simulink model "flight_sim"  (R2021b)
settings: Solver=ode45  StartTime=0.0  StopTime=300  RelTol=1e-3
values from neighbouring files (symbols this model uses):
  fpa_0 = pi/2    (= 1.57079632679)    [Falcon_1_para.m]
  fpa_in = 0.10    (= 0.1)    [Falcon_1_para.m]
  g = 9.81    [Falcon_1_para.m]
  h_0 = 0    [Falcon_1_para.m]
  m_dot = 132.46    [Falcon_1_para.m]
  m_zfw = m_pay + m_dry    (= 6360.7)    [Falcon_1_para.m]
  R_E = 6731e03    (= 6731000)    [Falcon_1_para.m]
  t_turn = 30.0    (= 30)    [Falcon_1_para.m]
  v_0 = 0.01    [Falcon_1_para.m]
  x_0 = 0    [Falcon_1_para.m]
undefined symbols (not defined in the file or in its folder): Earth, WGS84
libraries: aerolibfltsims x2, slpidlib x1, aerolibtransform2 x1, simulink x1
settings Model: Creator=hashi  LastModifiedBy=hashi

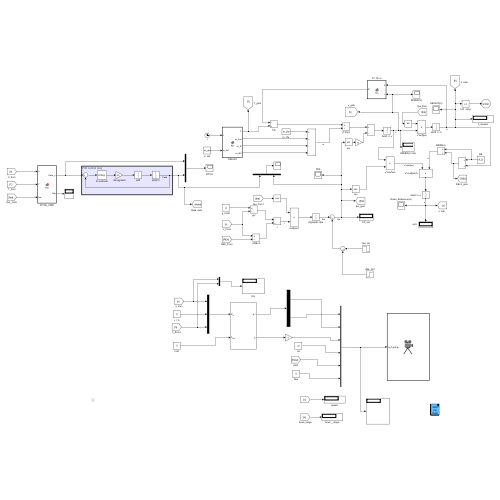
[thumbnail: Simulink's stored preview of the top-level diagram]
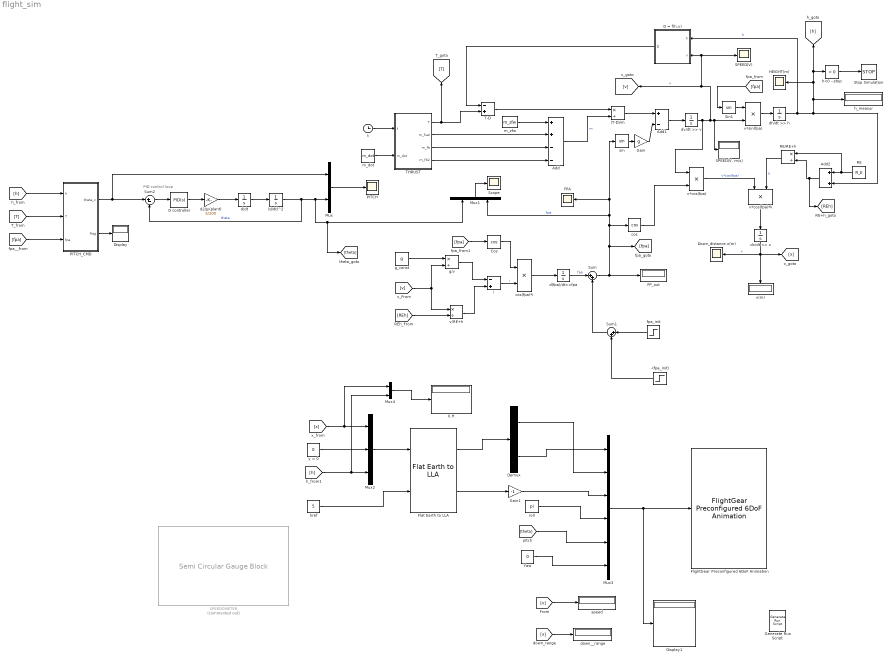
== system flight_sim ==
  note: PID control loop
  (T-D)/m : Product  Inputs=*/
  (d/dt)^2 : Integrator  InitialCondition=pi/2
  -(fpa_init) : Step  Time=t_turn+1  Before=-fpa_in  After=-fpa_in  SampleTime=0
  Add : Sum  Inputs=++--
  Add1 : Sum  Inputs=+-
  Add2 : Sum
  Cos : Trigonometry  Operator=cos
  D = f(h,v) : MATLAB Function  TreatAsAtomicUnit=on
  D controller : slpidlib/PID Controller  Controller=PID  Form=Parallel  TimeDomain=Continuous-time  UseExternalTs=off  SampleTime=-1  IntegratorMethod=Forward Euler  FilterMethod=Forward Euler  ControllerParametersSource=internal  P=0  I=0  D=200/5  UseFilter=on  N=100  TunerSelectOption=Transfer Function Based (PID Tuner App)  InitialConditionSource=internal  InitialConditionForIntegrator=0  InitialConditionForFilter=0  DifferentiatorICPrevScaledInput=0  ExternalReset=none  TrackingMode=off  Kt=1  LimitOutput=off  SatLimitsSource=internal  UpperSaturationLimit=inf  LowerSaturationLimit=-inf  LinearizeAsGain=on  AntiWindupMode=none  Kb=1  POutMin=[]  POutMax=[]  IOutMin=[]  IOutMax=[]  DOutMin=[]  DOutMax=[]  NOutMin=[]  NOutMax=[]  SumOutMin=[]  SumOutMax=[]  SaturationOutMin=[]  SaturationOutMax=[]  PParamMin=[]  PParamMax=[]  IParamMin=[]  IParamMax=[]  DParamMin=[]  DParamMax=[]  NParamMin=[]  NParamMax=[]  KbParamMin=[]  KbParamMax=[]  KtParamMin=[]  KtParamMax=[]  KbOutMin=[]  KbOutMax=[]  KtOutMin=[]  KtOutMax=[]  IntegratorOutMin=[]  IntegratorOutMax=[]  FilterOutMin=[]  FilterOutMax=[]  SumI1OutMin=[]  SumI1OutMax=[]  SumI2OutMin=[]  SumI2OutMax=[]  SumI3OutMin=[]  SumI3OutMax=[]  SumI4OutMin=[]  SumI4OutMax=[]  SumDOutMin=[]  SumDOutMax=[]  DifferentiatorOutMin=[]  DifferentiatorOutMax=[]  FilterDiffOutCoefMin=[]  FilterDiffOutCoefMax=[]  ReciprocalOutMin=[]  ReciprocalOutMax=[]  SumDenOutMin=[]  SumDenOutMax=[]  SumNumOutMin=[]  SumNumOutMax=[]  DivideOutMin=[]  DivideOutMax=[]  UdiffTsProdOutMin=[]  UdiffTsProdOutMax=[]  NTsProdOutMin=[]  NTsProdOutMax=[]  UintegralTsProdOutMin=[]  UintegralTsProdOutMax=[]  UngainTsProdOutMin=[]  UngainTsProdOutMax=[]  IntegratorContinuousStateAttributes=''  IntegratorStateMustResolveToSignalObject=off  IntegratorRTWStateStorageClass=Auto  FilterContinuousStateAttributes=''  FilterStateMustResolveToSignalObject=off  FilterRTWStateStorageClass=Auto  ParallelPVariant=InternalParameters  IdealPVariant=Disabled  IVariant=InternalParameters  DVariant=InternalParameters  IntegratorVariant=Continuous  SatVariant=Disabled  AWVariant=Passthrough  PCopyVariant=Disabled  TRVariant=Disabled  FdbkBlocksVariant=Forward  IdealPFdbkVariant=Disabled  SatFdbkVariant=Disabled  DerivativeFilterVariant=ContFilter  NVariant=InternalParameters  NCopyVariant=Disabled  FilterICVariant=InternalICsFilter  IntegratorICVariant=InternalICs  ExternalResetVariant=Disabled  TRSumVariant=Passthrough  SumFdbkVariant=Disabled  SumVariant=Sum_PID  TsampFilterVariant=InternalTs  TsampNgainVariant=Passthrough  TsampIntegralVariant=Passthrough  ExternalSaturationOutDataTypeStr=Inherit: Same as second input
  Demux : Demux  Outputs=2
  Display : Display
  Display1 : Display
  Down_distance,x(m) : Scope
  FPA : Scope
  FP_out : Display
  Flat Earth to LLA : aerolibtransform2/Flat Earth to LLA  units=Metric (MKS)  ptype=Earth (WGS84)  F=1/298.257223563  R=6378137  refPosPort=off  LL0=[28.608397 -80.604345]  psi=0
  FlightGear Preconfigured 6DoF Animation : aerolibfltsims/FlightGear Preconfigured 6DoF Animation  xFlightGearVersion=v2019.1  DestinationIpAddress=127.0.0.1  DestinationPort=5502  SampleTime=1/30  packetVersion=24
  Gain : Gain  Gain=g
  Gain1 : Gain  Gain=-1
  Generate Run Script : aerolibfltsims/Generate Run Script  Architecture=Win64  dataFlow=Send  GeometryModelName=rocket  AirportId=KSFO  RunwayId=10L  InitialAltitude=7224  InitialHeading=113  OffsetDistance=4.72  OffsetAzimuth=0  InstallScenery=on  DisableShaders=on  OriginAddress=127.0.0.1  DestinationPort=5502  OriginPort=5505  LocalAddress=127.0.0.1  OutputFileName=runfg.bat  FlightGearBaseDirectory=C:\Program Files\FlightGear 2020.3
  HEIGHT(m) : Scope
  Mux : Mux  Inputs=2
  Mux1 : Mux  Inputs=2
  Mux2 : Mux  Inputs=3
  Mux3 : Mux  Inputs=6
  Mux4 : Mux  Inputs=2
  PITCH : Scope
  PITCH_CMD : MATLAB Function  TreatAsAtomicUnit=on
  RE : Constant  Value=R_E
  RE/RE+h : Product  Inputs=*/
  SPEED(V) : Scope
  "SPEED(V, m/s)" : Display
  SPEEDOMETER : SemiCircularGaugeBlock  Commented=on
  Scope : Scope
  Sin1 : Trigonometry
  Stop Simulation : Stop
  Sum : Sum  Inputs=|++
  Sum1 : Sum  Inputs=|++
  Sum2 : Sum  Inputs=|+-
  T-D : Sum  Inputs=-+
  THRUST : MATLAB Function  TreatAsAtomicUnit=on
  X,H : Display
  Yaw : Constant  Value=0
  cos : Trigonometry  Operator=cos
  cos(fpa)*i : Product
  d(fpa)/dt>>fpa : Integrator  InitialCondition=fpa_0
  d/dt : Integrator
  d2/Jy(plant) : Gain  Gain=5/200
  dh/dt >> h : Integrator  InitialCondition=h_0
  down__range : Display
  dv/dt >> v : Integrator  InitialCondition=v_0
  dx/dt >> x : Integrator  InitialCondition=x_0
  fpa_init : Step  Time=t_turn  Before=fpa_in  After=0  SampleTime=0
  g/v : Product  Inputs=*/
  g_const : Constant  Value=g
  h<0 --stop : simulink/Logic and Bit Operations/Compare To Zero  relop=<  OutDataTypeStr=boolean
  h_measur : Display
  href : Constant  Value=5
  i : Sum  Inputs=-+
  m_dot : Constant  Value=m_dot
  m_zfw : Constant  Value=m_zfw
  roll : Constant  Value=pi
  sin : Trigonometry
  speed : Display
  t : Clock
  v*cos(fpa) : Product
  v*cos(fpa)*k : Product
  v*sin(fpa) : Product
  v/RE+h : Product  Inputs=*/
  x(m) : Display
  y = 0 : Constant  Value=0
  wires:
  m_dot/1 -> THRUST/2(m_dot)
  t/1 -> THRUST/1(t)
  m_zfw/1 -> Add/1
  THRUST/2(m_fuel) -> Add/2
  THRUST/3(m_fb) -> Add/3
  THRUST/4(m_fb2) -> Add/4
  T-D/1 -> (T-D)/m/1
  Add/1 -> (T-D)/m/2  "m"
  (T-D)/m/1 -> Add1/1
  Gain/1 -> Add1/2
  sin/1 -> Gain/1
  Add1/1 -> dv/dt >> v/1
  dv/dt >> v/1 -> v*cos(fpa)/1, "SPEED(V, m/s)"/1, v*sin(fpa)/2, SPEED(V)/1, D = f(h,v)/2(v), [v]  "v"
  v*sin(fpa)/1 -> dh/dt >> h/1
  dh/dt >> h/1 -> Add2/2, [h], h<0 --stop/1, HEIGHT(m)/1, h_measur/1, D = f(h,v)/1(h)  "h"
  D = f(h,v)/1(D) -> T-D/1
  h<0 --stop/1 -> Stop Simulation/1
  THRUST/1(T) -> T-D/2, [T]
  RE/1 -> Add2/1, RE/RE+h/1
  RE/RE+h/1 -> v*cos(fpa)*k/2  "k"
  v*cos(fpa)*k/1 -> dx/dt >> x/1
  dx/dt >> x/1 -> Down_distance,x(m)/1, [x], x(m)/1  "x"
  [REh] -> v/RE+h/2
  [v] -> v/RE+h/1, g/v/2
  g_const/1 -> g/v/1
  g/v/1 -> i/1
  v/RE+h/1 -> i/2
  i/1 -> cos(fpa)*i/2  "i"
  Cos/1 -> cos(fpa)*i/1
  cos(fpa)*i/1 -> d(fpa)/dt>>fpa/1
  d(fpa)/dt>>fpa/1 -> Sum/1  "fpa"
  cos/1 -> v*cos(fpa)/2
  v*cos(fpa)/1 -> v*cos(fpa)*k/1  "v*cos(fpa)"
  Sin1/1 -> v*sin(fpa)/1
  [fpa] -> Sin1/1
  fpa_init/1 -> Sum1/1
  -(fpa_init)/1 -> Sum1/2
  Sum1/1 -> Sum/2
  [h] -> PITCH_CMD/1(h)
  [T] -> PITCH_CMD/2(T)
  [fpa] -> PITCH_CMD/3(fpa)
  PITCH_CMD/2(flag) -> Display/1
  PITCH_CMD/1(theta_c) -> Mux/1, Sum2/1
  Sum2/1 -> D controller/1
  D controller/1 -> d2/Jy(plant)/1
  d2/Jy(plant)/1 -> d/dt/1
  d/dt/1 -> (d/dt)^2/1
  (d/dt)^2/1 -> Sum2/2, [theta], Mux1/1, Mux/2  "theta"
  Mux/1 -> PITCH/1
  Sum/1 -> FP_out/1, cos/1, Mux1/2, FPA/1, sin/1, [fpa]  "fpa"
  [fpa] -> Cos/1
  Add2/1 -> [REh], RE/RE+h/2
  Mux1/1 -> Scope/1
  Flat Earth to LLA/1 -> Demux/1
  Mux2/1 -> Flat Earth to LLA/1
  [x] -> Mux4/1, Mux2/1
  y = 0/1 -> Mux2/2
  [h] -> Mux4/2, Mux2/3
  href/1 -> Flat Earth to LLA/2
  Demux/1 -> Mux3/2
  Demux/2 -> Mux3/1
  Flat Earth to LLA/2 -> Gain1/1
  Gain1/1 -> Mux3/3
  roll/1 -> Mux3/4
  [theta] -> Mux3/5
  Yaw/1 -> Mux3/6
  Mux3/1 -> Display1/1, FlightGear Preconfigured 6DoF Animation/1
  [v] -> speed/1
  [x] -> down__range/1
  Mux4/1 -> X,H/1

== matlab function flight_sim/PITCH_CMD ==
  settings: updateMethod=DISCRETE
  data: h input; theta_c output; T input; fpa input; flag output
function [theta_c, flag] = fcn(h, T, fpa)

    persistent f % for flag output
    if isempty(f)
        f = 0;
    end    
  % Phase 2 begins if T<=0 and/or h <1000 m.
    if T<=0
        thet_c = fpa + pi;
        if thet_c>pi
            thet_c = pi;
        end
        f = 1; % now flag set to 1, whcih indicates the Phase 2 initiation
    elseif T<=0 && h<1000
        thet_c = pi/2; % perpendicular to the ground
    else
        thet_c = fpa; %Phase 1 condition
    end

    flag = f;
    theta_c = thet_c;

== matlab function flight_sim/THRUST ==
  settings: updateMethod=DISCRETE
  data: t input; T output; m_fuel output; m_fb output; m_fb2 output; m_dot input
function [T, m_fuel, m_fb, m_fb2] = fcn(t, m_dot)

    persistent mfb
    persistent mfb2

    if isempty(mfb)
        mfb=0;
    end
    if isempty(mfb2)
        mfb2=0;
    end

    mfuel = 21491.26; %Fuel Mass,kg

    %% Phase 1: TakeOff
    %Max thrust till 65% of fuel
    if mfb <=0.65*mfuel
        THRUST = 346961.28; %full thrust
        mfb = t*m_dot; % will get mass of fuel
    else
        THRUST = 0;
    end

    %% Boostback and Entry burn
    
    if (125<t) && (t<295)
        THRUST = -110000;
        mfb2 = (t-125)*(m_dot/3);
    end

    T = THRUST;
    m_fb = mfb;
    m_fb2 = mfb2;
    m_fuel = mfuel;

== matlab function flight_sim/D = f(h,v) ==
  data: h input; D output; v input
function D = fcn(h,v)
  
    Cd = 0.075; %Drag coeff
    Di = 1.5; %meter, diameter of launch vehicle(Vehicle model)
    A = pi*Di^2/4; % Area
    
    %% Earth Atmospheric model(ISA) for density

    if h<=11000
        T = 15.04-0.00649*h;
        p = 101.29*((T+273.1)/288.08)^5.258;
    elseif (11000<h) && (h<=25000)
        T = -56.46;
        p = 22.65*exp(1.73-0.000157*h);
    else 
        %h > 25000
        T = -131.21+0.00299*h;
        p = 2.488*((T+273.1)/216.6)^-11.388;
    end

    % Density
    rho = p / (0.2869*(T+273.1));

    %% Drag Force,D
    Drag = 0.5*Cd*rho*A*v^2;
    
    D = Drag;
